simulink model "AdaptiveControl"  (R2020b)
settings: Solver=VariableStepAuto  StartTime=0.0  StopTime=100  RelTol=1e-3
values from neighbouring files (symbols this model uses):
  F_initial = 0.7    [parameters.m]
  F_real = 1    [parameters.m]
  G_initial = 1.8    [parameters.m]
  G_real = 2    [parameters.m]
  I_initial = 0.5    [parameters.m]
  I_real = 1    [parameters.m]
  K_theta = eye(3,3)    [parameters.m]
  KD = 100    [parameters.m]
  lambda = 80    [parameters.m]
settings Model: Creator=Edoardo  LastModifiedBy=Edoardo

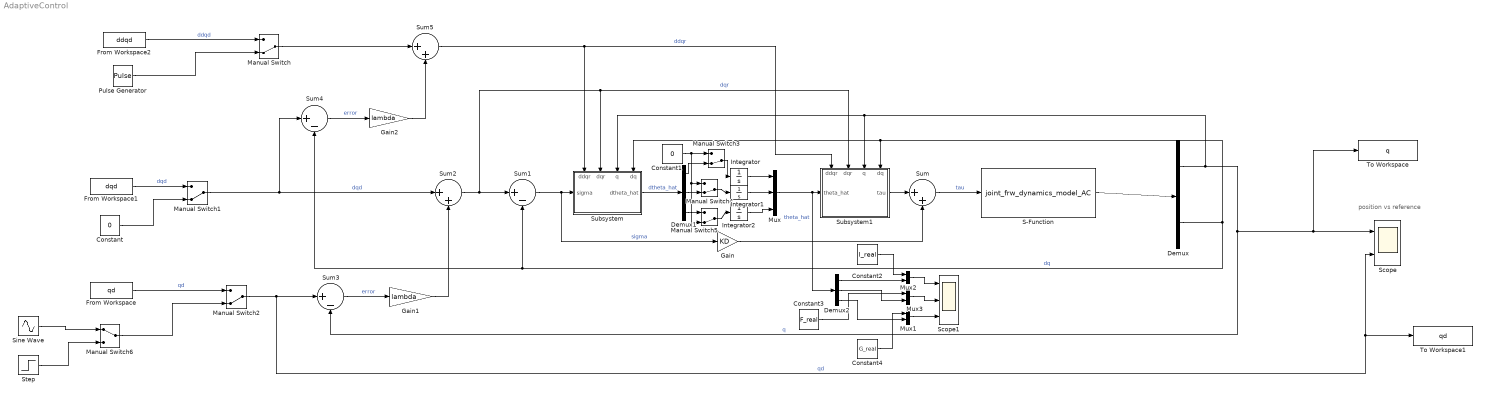
== system AdaptiveControl ==
  note: position vs reference
  Constant : Constant  Value=0
  Constant1 : Constant  Value=0
  Constant2 : Constant  Value=I_real
  Constant3 : Constant  Value=F_real
  Constant4 : Constant  Value=G_real
  Demux : Demux  Outputs=2
  Demux1 : Demux  Outputs=3
  Demux2 : Demux  Outputs=3
  From Workspace : FromWorkspace  VariableName=qd
  From Workspace1 : FromWorkspace  VariableName=dqd
  From Workspace2 : FromWorkspace  VariableName=ddqd
  Gain : Gain  Gain=KD
  Gain1 : Gain  Gain=lambda
  Gain2 : Gain  Gain=lambda
  Integrator : Integrator  InitialCondition=I_initial
  Integrator1 : Integrator  InitialCondition=F_initial
  Integrator2 : Integrator  InitialCondition=G_initial
  Manual Switch{,1..5} (6 alike) : ManualSwitch  CurrentSetting=0
  Manual Switch6 : ManualSwitch
  Mux : Mux  Inputs=3
  Mux1 : Mux  Inputs=2
  Mux2 : Mux  Inputs=2
  Mux3 : Mux  Inputs=2
  Pulse Generator : DiscretePulseGenerator  PulseType=Time based  Period=10  PulseWidth=5
  S-Function : S-Function  FunctionName=joint_frw_dynamics_model_AC  Parameters=myRobot  SFunctionDeploymentMode=off  EnableBusSupport=off
  Scope : Scope  NumInputPorts=2
  Scope1 : Scope  NumInputPorts=3
  Sine Wave : Sin  SampleTime=0
  Step : Step  SampleTime=0
  Subsystem : Subsystem
      settings: PortSchema="{\"entries\":[{\"content\":{\"sides\":[{\"content\":{\"connectorIds\":[\"In1\"]},\"type\":\"ConnectorPlacement.EquallySpacedRectSide\",\"uuid\":\"4a8d65ed-741d-467f-8b00-988d92c9f269\"},{\"content\":{\"connectorIds\":[\"Out1\"],\"side\":\"RIGHT\"},\"type\":\"ConnectorPlacement.EquallySpacedRectSide\",\"uuid\":\"f96a52d3-c8a1-4150-b1ce-025da4f2b639\"},{\"content\":{\"connectorIds\":[\"In2\",\"In3\",\"In4\",\"In5\"],\"side\":\"TOP\"},\"type\":\"ConnectorPlacement.EquallySpacedRectSide\",\"uuid\":\"fe0bae09-66a3-4a77-8685-5eeef3c108a2\"},{\"content\":{\"connectorIds\":[],\"side\":\"HIDDEN\"},\"type\":\"ConnectorPlacement.EquallySpacedRectSide\",\"uuid\":\"d6c670c3-faf9-4599-babb-26cc4d3984ba\"}]},\"type\":\"ConnectorPlacement.EquallySpacedConnector\",\"uuid\":\"66a62a24-f35c-4704-8912-2a8fcfa51c4e\"}],\"packageUris\":[\"http://schema.mathworks.com/mf0/Connector/R2020b\"],\"version\":\"1.0\"}"
  Subsystem1 : Subsystem
      settings: PortSchema="{\"entries\":[{\"content\":{\"sides\":[{\"content\":{\"connectorIds\":[\"In1\"]},\"type\":\"ConnectorPlacement.EquallySpacedRectSide\",\"uuid\":\"4a8d65ed-741d-467f-8b00-988d92c9f269\"},{\"content\":{\"connectorIds\":[\"Out1\"],\"side\":\"RIGHT\"},\"type\":\"ConnectorPlacement.EquallySpacedRectSide\",\"uuid\":\"f96a52d3-c8a1-4150-b1ce-025da4f2b639\"},{\"content\":{\"connectorIds\":[\"In2\",\"In3\",\"In4\",\"In5\"],\"side\":\"TOP\"},\"type\":\"ConnectorPlacement.EquallySpacedRectSide\",\"uuid\":\"fe0bae09-66a3-4a77-8685-5eeef3c108a2\"},{\"content\":{\"connectorIds\":[],\"side\":\"HIDDEN\"},\"type\":\"ConnectorPlacement.EquallySpacedRectSide\",\"uuid\":\"d6c670c3-faf9-4599-babb-26cc4d3984ba\"}]},\"type\":\"ConnectorPlacement.EquallySpacedConnector\",\"uuid\":\"66a62a24-f35c-4704-8912-2a8fcfa51c4e\"}],\"packageUris\":[\"http://schema.mathworks.com/mf0/Connector/R2020b\"],\"version\":\"1.0\"}"
  Sum : Sum  Inputs=|++
  Sum1 : Sum  Inputs=|+-
  Sum2 : Sum  Inputs=|++
  Sum3 : Sum  Inputs=|+-
  Sum4 : Sum  Inputs=|+-
  Sum5 : Sum  Inputs=|++
  To Workspace : ToWorkspace  VariableName=q  SaveFormat=Timeseries  SampleTime=-1
  To Workspace1 : ToWorkspace  VariableName=qd  SaveFormat=Timeseries  SampleTime=-1
  wires:
  S-Function/1 -> Demux/1
  Sum/1 -> S-Function/1  "tau"
  Subsystem1/1(tau) -> Sum/1
  Mux/1 -> Demux2/1, Subsystem1/1(theta_hat)  "theta_hat"
  Subsystem/1(dtheta_hat) -> Demux1/1  "dtheta_hat"
  Gain/1 -> Sum/2
  Sum1/1 -> Subsystem/1(sigma), Gain/1  "sigma"
  Sum2/1 -> Subsystem1/3(dqr), Subsystem/3(dqr), Sum1/1  "dqr"
  Gain1/1 -> Sum2/2
  Sum3/1 -> Gain1/1  "error"
  Manual Switch2/1 -> To Workspace1/1, Scope/2, Sum3/1  "qd"
  Manual Switch1/1 -> Sum2/1, Sum4/1  "dqd"
  Sum4/1 -> Gain2/1  "error"
  Gain2/1 -> Sum5/2
  Demux/1 -> Sum3/2, To Workspace/1, Scope/1, Subsystem/4(q), Subsystem1/4(q)  "q"
  Demux/2 -> Subsystem/5(dq), Subsystem1/5(dq), Sum1/2, Sum4/2  "dq"
  Sum5/1 -> Subsystem1/2(ddqr), Subsystem/2(ddqr)  "ddqr"
  Manual Switch/1 -> Sum5/1
  From Workspace/1 -> Manual Switch2/1  "qd"
  From Workspace1/1 -> Manual Switch1/1  "dqd"
  From Workspace2/1 -> Manual Switch/1  "ddqd"
  Manual Switch6/1 -> Manual Switch2/2
  Pulse Generator/1 -> Manual Switch/2
  Constant/1 -> Manual Switch1/2
  Integrator/1 -> Mux/1
  Integrator1/1 -> Mux/2
  Integrator2/1 -> Mux/3
  Demux1/2 -> Manual Switch4/2
  Manual Switch4/1 -> Integrator1/1
  Manual Switch3/1 -> Integrator/1
  Demux1/1 -> Manual Switch3/2
  Manual Switch5/1 -> Integrator2/1
  Demux1/3 -> Manual Switch5/2
  Constant1/1 -> Manual Switch5/1, Manual Switch4/1, Manual Switch3/1
  Sine Wave/1 -> Manual Switch6/1
  Step/1 -> Manual Switch6/2
  Demux2/1 -> Mux2/2
  Demux2/2 -> Mux3/2
  Demux2/3 -> Mux1/2
  Mux2/1 -> Scope1/1
  Mux3/1 -> Scope1/2
  Constant4/1 -> Mux1/1
  Constant3/1 -> Mux3/1
  Constant2/1 -> Mux2/1
  Mux1/1 -> Scope1/3

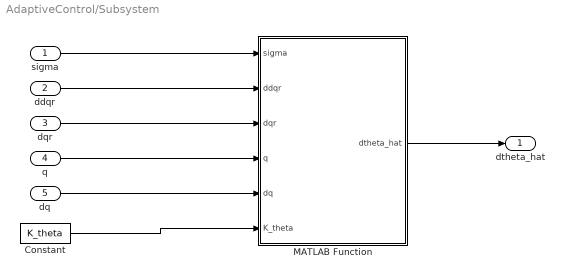
== system AdaptiveControl/Subsystem ==
  sigma : Inport
  ddqr : Inport  Port=2
  dqr : Inport  Port=3
  q : Inport  Port=4
  dq : Inport  Port=5
  Constant : Constant  Value=K_theta
  MATLAB Function : MATLAB Function  TreatAsAtomicUnit=on
  dtheta_hat : Outport
  wires:
  MATLAB Function/1(dtheta_hat) -> dtheta_hat/1
  sigma/1 -> MATLAB Function/1(sigma)
  ddqr/1 -> MATLAB Function/2(ddqr)
  dqr/1 -> MATLAB Function/3(dqr)
  q/1 -> MATLAB Function/4(q)
  dq/1 -> MATLAB Function/5(dq)
  Constant/1 -> MATLAB Function/6(K_theta)

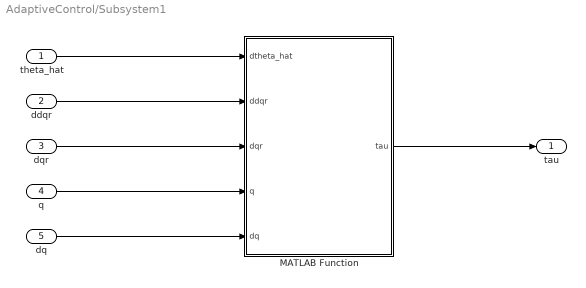
== system AdaptiveControl/Subsystem1 ==
  theta_hat : Inport
  ddqr : Inport  Port=2
  dqr : Inport  Port=3
  q : Inport  Port=4
  dq : Inport  Port=5
  MATLAB Function : MATLAB Function  TreatAsAtomicUnit=on
  tau : Outport
  wires:
  theta_hat/1 -> MATLAB Function/1(dtheta_hat)
  ddqr/1 -> MATLAB Function/2(ddqr)
  dqr/1 -> MATLAB Function/3(dqr)
  q/1 -> MATLAB Function/4(q)
  dq/1 -> MATLAB Function/5(dq)
  MATLAB Function/1(tau) -> tau/1

== matlab function AdaptiveControl/Subsystem1/MATLAB Function ==
  data: dtheta_hat input; tau output; ddqr input; dqr input; q input; dq input
function tau = compute_tau(dtheta_hat, ddqr, dqr, q, dq)
    
    Y = [ddqr, dqr, sin(q)];
    tau = Y*dtheta_hat;

== matlab function AdaptiveControl/Subsystem/MATLAB Function ==
  data: sigma input; dtheta_hat output; ddqr input; dqr input; q input; dq input; K_theta input
function dtheta_hat = compute_dtheta_hat(sigma, ddqr, dqr, q, dq, K_theta)
    
    Y = [ddqr, dqr, sin(q)];
    dtheta_hat = inv(K_theta)*Y'*sigma;
%dtheta_hat = 1;
